simulink model "simu_1"  (R2021a)
settings: Solver=VariableStepAuto  StartTime=0.0  StopTime=10.0  RelTol=1e-3
values from neighbouring files (symbols this model uses):
  b = 0.5    [clase_2.mat]
  k = 2    [clase_2.mat]
  m = 1    [clase_2.mat]
settings Model: Creator=pierr  LastModifiedBy=pierr

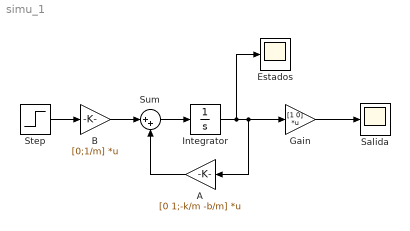
== system simu_1 ==
  A : Gain  Gain=[0 1;-k/m -b/m]  Multiplication=Matrix(K*u)
  B : Gain  Gain=[0;1/m]  Multiplication=Matrix(K*u)
  Estados : Scope
  Gain : Gain  Gain=[1 0]  Multiplication=Matrix(K*u)
  Integrator : Integrator
  Salida : Scope
  Step : Step  Time=0  SampleTime=0
  Sum : Sum  Inputs=|++
  wires:
  Step/1 -> B/1
  A/1 -> Sum/2
  B/1 -> Sum/1
  Integrator/1 -> Estados/1, A/1, Gain/1
  Sum/1 -> Integrator/1
  Gain/1 -> Salida/1
